simulink model "controller1"  (R2022a)
settings: Solver=VariableStepAuto  StartTime=0.0  StopTime=44  MaxStep=1e-3  MinStep=1e-6  RelTol=1e-3
libraries: dspswit3 x1
(part 1 of 2)
settings Model: Creator=LALO  LastModifiedBy=LALO

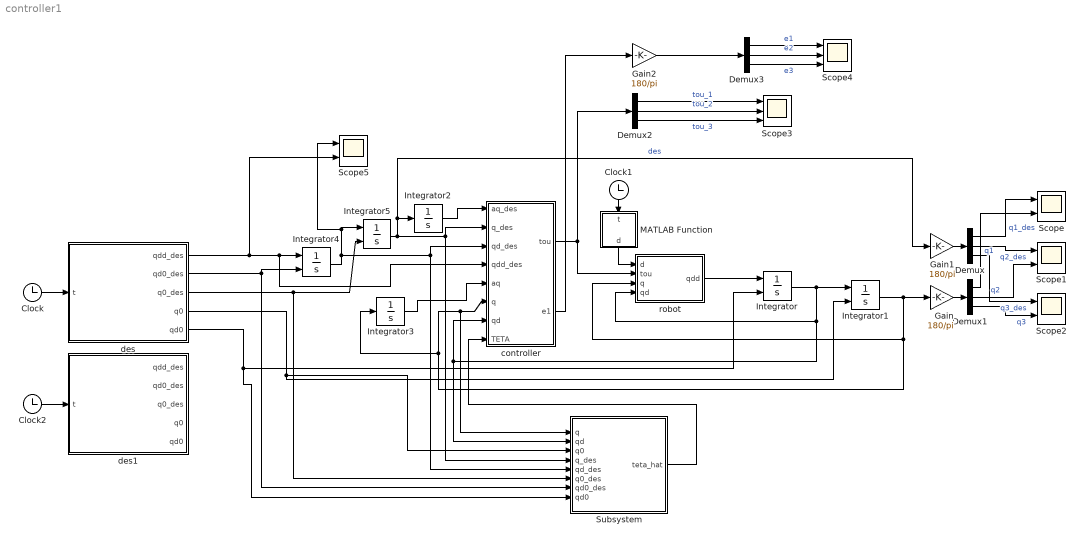
== system controller1 ==
  Clock : Clock
  Clock1 : Clock
  Clock2 : Clock
  Demux{,1..3} (4 alike) : Demux  Outputs=3
  Gain : Gain  Gain=180/pi
  Gain1 : Gain  Gain=180/pi
  Gain2 : Gain  Gain=180/pi
  Integrator{,1,4..5} (4 alike) : Integrator  InitialConditionSource=external
  Integrator2 : Integrator
  Integrator3 : Integrator
  MATLAB Function : MATLAB Function  TreatAsAtomicUnit=on
  Scope{,1..2,5} (4 alike) : Scope  NumInputPorts=2
  Scope3 : Scope  NumInputPorts=3
  Scope4 : Scope  NumInputPorts=3
  Subsystem : Subsystem
  controller : MATLAB Function  TreatAsAtomicUnit=on
  des : MATLAB Function  TreatAsAtomicUnit=on
  des1 : MATLAB Function  TreatAsAtomicUnit=on
  robot : MATLAB Function  TreatAsAtomicUnit=on
  wires:
  Clock/1 -> des/1(t)
  Integrator5/1 -> Subsystem/4(q_des), controller/2(q_des), Gain1/1, Integrator2/1  "des"
  des/1(qdd_des) -> Scope5/2, Integrator4/1, controller/4(qdd_des)
  robot/1(qdd) -> Integrator/1
  Integrator/1 -> robot/4(qd), Subsystem/2(qd), controller/7(qd), Integrator1/1
  Integrator1/1 -> Gain/1, robot/3(q), Subsystem/1(q), controller/6(q), Integrator3/1
  des/4(q0) -> Integrator1/2, Subsystem/3(q0)
  des/5(qd0) -> Subsystem/8(qd0), Integrator/2
  Clock1/1 -> MATLAB Function/1(t)
  MATLAB Function/1(d) -> robot/1(d)
  Integrator2/1 -> controller/1(aq_des)
  Integrator3/1 -> controller/5(aq)
  Integrator4/1 -> Scope5/1, Integrator5/1, Subsystem/5(qd_des), controller/3(qd_des)
  des/2(qd0_des) -> Integrator4/2, Subsystem/7(qd0_des)
  des/3(q0_des) -> Subsystem/6(q0_des), Integrator5/2
  Subsystem/1(teta_hat) -> controller/8(TETA)
  Gain1/1 -> Demux/1
  Gain/1 -> Demux1/1
  Demux/1 -> Scope/1  "q1_des"
  Demux/2 -> Scope1/1  "q2_des"
  Demux/3 -> Scope2/1  "q3_des"
  Demux1/1 -> Scope/2  "q1"
  Demux1/2 -> Scope1/2  "q2"
  Demux1/3 -> Scope2/2  "q3"
  Demux2/1 -> Scope3/1  "tou_1"
  Demux2/2 -> Scope3/2  "tou_2"
  Demux2/3 -> Scope3/3  "tou_3"
  controller/1(tou) -> robot/2(tou), Demux2/1
  Demux3/1 -> Scope4/1  "e1"
  Demux3/3 -> Scope4/3  "e3"
  Demux3/2 -> Scope4/2  "e2"
  Clock2/1 -> des1/1(t)
  Gain2/1 -> Demux3/1
  controller/2(e1) -> Gain2/1

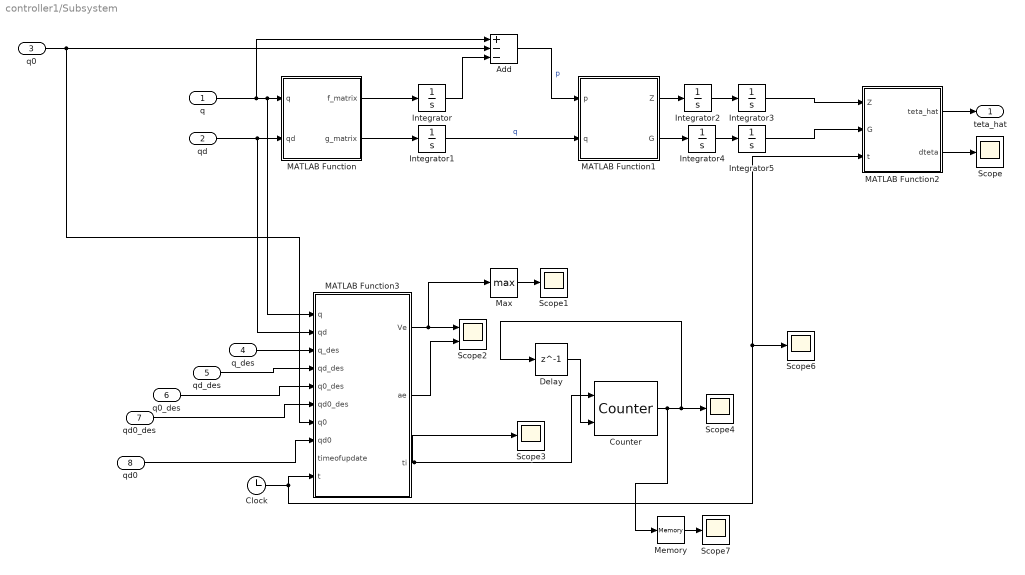
== system controller1/Subsystem ==
  q : Inport
  qd : Inport  Port=2
  q0 : Inport  Port=3
  q_des : Inport  Port=4
  qd_des : Inport  Port=5
  q0_des : Inport  Port=6
  qd0_des : Inport  Port=7
  qd0 : Inport  Port=8
  Add : Sum  Inputs=+--
  Clock : Clock
  Counter : dspswit3/Counter  Direction=Up  CountEvent=Rising edge  CounterSize=User defined  MaxCount=255  InitialCount=0  Output=Count  HitValue=1  ResetInput=on  SamplesPerFrame=1  Ts=1  CntDtype=double  HitDtype=Boolean
  Delay : Delay  DelayLength=1
  Integrator{,1..5} (6 alike) : Integrator
  MATLAB Function : MATLAB Function  TreatAsAtomicUnit=on
  MATLAB Function1 : MATLAB Function  TreatAsAtomicUnit=on
  MATLAB Function2 : MATLAB Function  TreatAsAtomicUnit=on
  MATLAB Function3 : MATLAB Function  TreatAsAtomicUnit=on
  Max : MinMax  Function=max
  Memory : Memory
  Scope{,1,3..4,6..7} (6 alike) : Scope
  Scope2 : Scope  NumInputPorts=2
  teta_hat : Outport
  wires:
  q/1 -> Add/1, MATLAB Function3/1(q), MATLAB Function/1(q)
  qd/1 -> MATLAB Function3/2(qd), MATLAB Function/2(qd)
  q0/1 -> MATLAB Function3/7(q0), Add/2
  MATLAB Function/1(f_matrix) -> Integrator/1
  MATLAB Function/2(g_matrix) -> Integrator1/1
  Integrator/1 -> Add/3
  Add/1 -> MATLAB Function1/1(p)  "p"
  Integrator1/1 -> MATLAB Function1/2(q)  "q"
  MATLAB Function1/1(Z) -> Integrator2/1
  Integrator2/1 -> Integrator3/1
  MATLAB Function1/2(G) -> Integrator4/1
  Integrator4/1 -> Integrator5/1
  q_des/1 -> MATLAB Function3/3(q_des)
  qd_des/1 -> MATLAB Function3/4(qd_des)
  MATLAB Function3/1(Ve) -> Max/1, Scope2/1
  MATLAB Function3/2(ae) -> Scope2/2
  Clock/1 -> Scope6/1, MATLAB Function2/3(t), MATLAB Function3/10(t)
  q0_des/1 -> MATLAB Function3/5(q0_des)
  qd0_des/1 -> MATLAB Function3/6(qd0_des)
  qd0/1 -> MATLAB Function3/8(qd0)
  MATLAB Function3/3(ti) -> Scope3/1, Counter/1
  Counter/1 -> Memory/1, Delay/1, Scope4/1
  Delay/1 -> Counter/2
  Memory/1 -> Scope7/1
  MATLAB Function2/1(teta_hat) -> teta_hat/1
  MATLAB Function2/2(dteta) -> Scope/1
  Integrator3/1 -> MATLAB Function2/1(Z)
  Integrator5/1 -> MATLAB Function2/2(G)
  Max/1 -> Scope1/1

== matlab function controller1/des1 ==
  data: t input; qdd_des output; qd0_des output; q0_des output; q0 output; qd0 output
function [qdd_des,qd0_des,q0_des,q0,qd0] = fcn(t)
q0=[pi/30;pi/35;pi/20];
qd0=[0;0;0];

% q0_des=[(80*pi/180);0;(25*pi/180)];
% qd0_des=[0;-(25*pi/180);0];
% qdd_des=[-(80*pi/180)*cos(t);(25*pi/180)*sin(t);-(25*pi/180)*cos(t)];
q0_des=[0;0;0];
qd0_des=[0;0;0];
qdd_des=[0;0;((-40*6/13.5)*t+(80/3))*pi/180];

if t>3

qdd_des=[((-90*6/32)*(t-3)+(33.75))*pi/180;0;0];
end

if t>7
qdd_des=[0;0;((40*6/13.5)*(t-7)+(-80/3))*pi/180];
end

if t>10
qdd_des=[0;((-70*6/13.5)*(t-10)+(140/3))*pi/180;0];
end

if t>13
qdd_des=[((90*6/32)*(t-13)+(-33.75))*pi/180;0;0];
end

if t>17
    qdd_des=[0;((70*6/13.5)*(t-17)+(-140/3))*pi/180;0];
end


if t>20
qdd_des=[0;0;((-40*6/13.5)*(t-20)+(80/3))*pi/180];
end

if t>23

qdd_des=[((-90*6/32)*(t-23)+(33.75))*pi/180;0;0];
end

if t>27
qdd_des=[0;0;((40*6/13.5)*(t-27)+(-80/3))*pi/180];
end

if t>30
qdd_des=[0;((-70*6/13.5)*(t-30)+(140/3))*pi/180;0];
end

if t>33
qdd_des=[((90*6/32)*(t-33)+(-33.75))*pi/180;0;0];
end

if t>37
    qdd_des=[0;((70*6/13.5)*(t-37)+(-140/3))*pi/180;0];
end

== matlab function controller1/robot ==
  data: d input; tou input; qdd output; q input; qd input
function qdd = fcn(d,tou,q,qd)
% q1=q(1);
q2=q(2);
q3=q(3);
dq1=qd(1);
dq2=qd(2);
dq3=qd(3);

Izz1=0.192;
Ixx3=0.063; Iyy3=0.061; Izz3= 0.02;
Ixx2=0.0027; Iyy2=0.0024; Izz2=0.0004;
%
M =[Izz1 + Ixx2*cos(q2)^2 + Iyy2*sin(q2)^2 + Izz3*sin(q2)^2 + Ixx3*cos(q2)^2*cos(q3)^2 + Iyy3*cos(q2)^2*sin(q3)^2,         cos(q2)*cos(q3)*sin(q3)*(Ixx3 - Iyy3), Izz3*sin(q2)
                                                                        cos(q2)*cos(q3)*sin(q3)*(Ixx3 - Iyy3), Iyy3 + Izz2 + Ixx3*sin(q3)^2 - Iyy3*sin(q3)^2,            0
                                                                                                 Izz3*sin(q2),                                             0,         Izz3];
 

C =[                                                                                                -(dq1*(Ixx3*sin(2*q2 + 2*q3) - Iyy3*sin(2*q2 + 2*q3) + 2*Ixx2*sin(2*q2) + Ixx3*sin(2*q2) + Ixx3*sin(2*q3) - 2*Iyy2*sin(2*q2) + Iyy3*sin(2*q2) - Iyy3*sin(2*q3) - 2*Izz3*sin(2*q2)))/4, -(dq1*cos(q2)*(Ixx3 - Iyy3 + Izz3 - 2*Ixx2*sin(q2) + 2*Iyy2*sin(q2) - 2*Iyy3*sin(q2) + 2*Izz3*sin(q2) - 2*Ixx3*cos(q3)^2 + 2*Iyy3*cos(q3)^2 - 2*Ixx3*cos(q3)^2*sin(q2) + 2*Iyy3*cos(q3)^2*sin(q2)))/2, (dq1*cos(q2)*(Ixx3 - Iyy3 + Izz3 - 2*Ixx3*cos(q3)^2 + 2*Iyy3*cos(q3)^2 + 2*Ixx3*cos(q2)*cos(q3)*sin(q3) - 2*Iyy3*cos(q2)*cos(q3)*sin(q3)))/2
(dq2*(2*Izz3*cos(q2) - 2*Ixx2*sin(2*q2) - Ixx3*sin(2*q2) + 2*Iyy2*sin(2*q2) - Iyy3*sin(2*q2) + 2*Izz3*sin(2*q2) - Ixx3*cos(2*q3)*sin(2*q2) + Iyy3*cos(2*q3)*sin(2*q2) + 2*Ixx3*cos(2*q3)*cos(q2) - 2*Iyy3*cos(2*q3)*cos(q2) - 2*Ixx3*sin(2*q3)*sin(q2) + 2*Iyy3*sin(2*q3)*sin(q2)))/4,                                                                                                                                                                       (dq2*sin(2*q3)*(Ixx3 - Iyy3))/2, (dq2*(Ixx3*cos(q2) - Iyy3*cos(q2) + Izz3*cos(q2) - Ixx3*sin(2*q3) + Iyy3*sin(2*q3) - 2*Ixx3*cos(q2)*cos(q3)^2 + 2*Iyy3*cos(q2)*cos(q3)^2))/2
                                                                                                                                         (dq3*cos(q2)*(Iyy3 - Ixx3 + Izz3 + 2*Ixx3*cos(q3)^2 - 2*Iyy3*cos(q3)^2 - 2*Ixx3*cos(q2)*cos(q3)*sin(q3) + 2*Iyy3*cos(q2)*cos(q3)*sin(q3)))/2,                                                         -(dq3*(Ixx3*cos(q2) - Iyy3*cos(q2) + Izz3*cos(q2) - Ixx3*sin(2*q3) + Iyy3*sin(2*q3) - 2*Ixx3*cos(q2)*cos(q3)^2 + 2*Iyy3*cos(q2)*cos(q3)^2))/2,                                                                                                                                            0];
 
G=[0;0;0];


qdd=M\(tou+d-C*qd-G);

== matlab function controller1/controller ==
  data: aq_des input; q_des input; tou output; qd_des input; qdd_des input; aq input; q input; qd input; TETA input; e1 output
function [tou,e1]  = fcn(aq_des,q_des,qd_des,qdd_des,aq,q,qd,TETA)
% q1=q(1);
q2=q(2);
q3=q(3);
dq1=qd(1);
dq2=qd(2);
dq3=qd(3);

% Ixx1=0.077; Iyy1=0.119;
% Izz1=0.192;
% Ixx3=0.063; Iyy3=0.061; Izz3= 0.02;
% Ixx2=0.0027; Iyy2=0.0024; Izz2=0.0004;
% Izz1=0.292;
% Ixx3=0.583; Iyy3=0.961; Izz3= 0.002;
% Ixx2=0.0017; Iyy2=0.0034; Izz2=0.0014;
Iyy3=(TETA(3)*TETA(1)^2/TETA(2)^2)^(1/3);
Ixx2=TETA(1)/Iyy3^2;
Izz3=(TETA(2)/TETA(1))*Iyy3;
Ixx3=TETA(5)/(Ixx2*Izz3);
Iyy2=TETA(6)/(Ixx3*Izz3);
Izz2=TETA(7)/(Izz3*Iyy2);
Izz1=TETA(4)/(Iyy3*Izz2);

% g=9.81;
ae1=aq-aq_des;
e1=q-q_des;
e2=qd-qd_des;
alfa=[8,0,0
      0,1,0
      0,0,4]*2;
beta=[1,0,0
      0,1,0
      0,0,2]*0.2;
gama=[1,0,0
      0,3,0
      0,0,1]*15;

%
M =[Izz1 + Ixx2*cos(q2)^2 + Iyy2*sin(q2)^2 + Izz3*sin(q2)^2 + Ixx3*cos(q2)^2*cos(q3)^2 + Iyy3*cos(q2)^2*sin(q3)^2,         cos(q2)*cos(q3)*sin(q3)*(Ixx3 - Iyy3), Izz3*sin(q2)
                                                                        cos(q2)*cos(q3)*sin(q3)*(Ixx3 - Iyy3), Iyy3 + Izz2 + Ixx3*sin(q3)^2 - Iyy3*sin(q3)^2,            0
                                                                                                 Izz3*sin(q2),                                             0,         Izz3];
 

C =[                                                                                                -(dq1*(Ixx3*sin(2*q2 + 2*q3) - Iyy3*sin(2*q2 + 2*q3) + 2*Ixx2*sin(2*q2) + Ixx3*sin(2*q2) + Ixx3*sin(2*q3) - 2*Iyy2*sin(2*q2) + Iyy3*sin(2*q2) - Iyy3*sin(2*q3) - 2*Izz3*sin(2*q2)))/4, -(dq1*cos(q2)*(Ixx3 - Iyy3 + Izz3 - 2*Ixx2*sin(q2) + 2*Iyy2*sin(q2) - 2*Iyy3*sin(q2) + 2*Izz3*sin(q2) - 2*Ixx3*cos(q3)^2 + 2*Iyy3*cos(q3)^2 - 2*Ixx3*cos(q3)^2*sin(q2) + 2*Iyy3*cos(q3)^2*sin(q2)))/2, (dq1*cos(q2)*(Ixx3 - Iyy3 + Izz3 - 2*Ixx3*cos(q3)^2 + 2*Iyy3*cos(q3)^2 + 2*Ixx3*cos(q2)*cos(q3)*sin(q3) - 2*Iyy3*cos(q2)*cos(q3)*sin(q3)))/2
(dq2*(2*Izz3*cos(q2) - 2*Ixx2*sin(2*q2) - Ixx3*sin(2*q2) + 2*Iyy2*sin(2*q2) - Iyy3*sin(2*q2) + 2*Izz3*sin(2*q2) - Ixx3*cos(2*q3)*sin(2*q2) + Iyy3*cos(2*q3)*sin(2*q2) + 2*Ixx3*cos(2*q3)*cos(q2) - 2*Iyy3*cos(2*q3)*cos(q2) - 2*Ixx3*sin(2*q3)*sin(q2) + 2*Iyy3*sin(2*q3)*sin(q2)))/4,                                                                                                                                                                       (dq2*sin(2*q3)*(Ixx3 - Iyy3))/2, (dq2*(Ixx3*cos(q2) - Iyy3*cos(q2) + Izz3*cos(q2) - Ixx3*sin(2*q3) + Iyy3*sin(2*q3) - 2*Ixx3*cos(q2)*cos(q3)^2 + 2*Iyy3*cos(q2)*cos(q3)^2))/2
                                                                                                                                         (dq3*cos(q2)*(Iyy3 - Ixx3 + Izz3 + 2*Ixx3*cos(q3)^2 - 2*Iyy3*cos(q3)^2 - 2*Ixx3*cos(q2)*cos(q3)*sin(q3) + 2*Iyy3*cos(q2)*cos(q3)*sin(q3)))/2,                                                         -(dq3*(Ixx3*cos(q2) - Iyy3*cos(q2) + Izz3*cos(q2) - Ixx3*sin(2*q3) + Iyy3*sin(2*q3) - 2*Ixx3*cos(q2)*cos(q3)^2 + 2*Iyy3*cos(q2)*cos(q3)^2))/2,                                                                                                                                            0];
 
G=[0;0;0];
%

h=qdd_des+M\(C*qd_des+G+C*e2);
tou=M*(h-(eye(3,3)+gama+beta*alfa)*e1-(alfa+beta)*e2-gama*ae1);
if tou(3)>0.9
tou(3)=0.9;
end
% if tou(1)>0.9
% tou(1)=0.9;
% end
% if tou(2)>0.9
% tou(2)=0.9;
% end

== matlab function controller1/des ==
  data: t input; qdd_des output; qd0_des output; q0_des output; q0 output; qd0 output
function [qdd_des,qd0_des,q0_des,q0,qd0] = fcn(t)
q0=[pi/30;pi/35;pi/20];
qd0=[0;0;0];

% q0_des=[(80*pi/180);0;(25*pi/180)];
% qd0_des=[0;-(25*pi/180);0];
% qdd_des=[-(80*pi/180)*cos(t);(25*pi/180)*sin(t);-(25*pi/180)*cos(t)];
q0_des=[0;0;0];
qd0_des=[0;0;0];
a=-10;
b=30;
T=t;
qdd_des=[0;0;((6*a)*(T)+(2*b))*pi/180];

if t>2
a= 5/2;
b=-15;
T=t-2;
qdd_des=[0;0;((6*a)*(T)+(2*b))*pi/180];
end
if t>6
a=-10;
b=30;
T=t-6;
qdd_des=[0;0;((6*a)*(T)+(2*b))*pi/180];
end

if t>8
a=-140/27;
b= 70/3;
T=t-8;
qdd_des=[0;((6*a)*(T)+(2*b))*pi/180;0];
end
if t>11
a=35/27;
b= -35/3;
T=t-11;
qdd_des=[0;((6*a)*(T)+(2*b))*pi/180;0];
end
if t>17
a=-140/27;
b= 70/3;
T=t-17;
qdd_des=[0;((6*a)*(T)+(2*b))*pi/180;0];
end

if t>20
a=-45/4;
b=135/4;
T=t-20;
qdd_des=[((6*a)*(T)+(2*b))*pi/180;0;0];
end

if t>22
a=-10;
b=30;
T=t-22;
qdd_des=[0;0;((6*a)*(T)+(2*b))*pi/180];
end
if t>24
a= 5/2;
b=-15;
T=t-24;
qdd_des=[0;0;((6*a)*(T)+(2*b))*pi/180];
end
if t>28
a=-10;
b=30;
T=t-28;
qdd_des=[0;0;((6*a)*(T)+(2*b))*pi/180];
end

if t>30
a=-140/27;
b= 70/3;
T=t-30;
qdd_des=[0;((6*a)*(T)+(2*b))*pi/180;0];
end
if t>33
a=35/27;
b= -35/3;
T=t-33;
qdd_des=[0;((6*a)*(T)+(2*b))*pi/180;0];
end
if t>39
a=-140/27;
b= 70/3;
T=t-39;
qdd_des=[0;((6*a)*(T)+(2*b))*pi/180;0];
end

if t>42
a=45/4;
b=-135/4;
T=t-42;
qdd_des=[((6*a)*(T)+(2*b))*pi/180;0;0];
end
end

== matlab function controller1/MATLAB Function ==
  data: t input; d output
function d= fcn(t)
d=[0;0;0];
if 13<t 
d=[0.05*sin(t-13)
    0.1
0.021];
end
if 21<t 
d=[0.2
    0.05
0.0];
end
if 25<t 
d=[0
   0
0.0];
end
